simulink model "model1"  (R2021b)
settings: Solver=VariableStepAuto  StartTime=0.0  StopTime=T_end  RelTol=1e-3
values from neighbouring files (symbols this model uses):
  Te = 0.1    [ex1.m]    (also in ex3.m; ex4.m; ex5.m; ex6.m)
  u_sat = 0.5    [ex1.m]    (also in ex3.m; ex4.m; ex5.m; ex6.m)
settings Model: Creator=Michael Biselx  LastModifiedBy=Michael Biselx

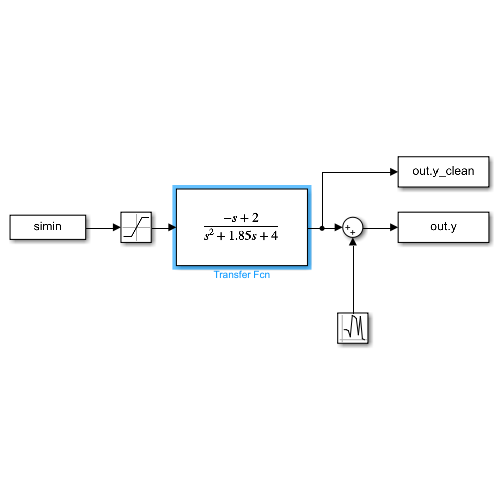
[thumbnail: Simulink's stored preview of the top-level diagram]
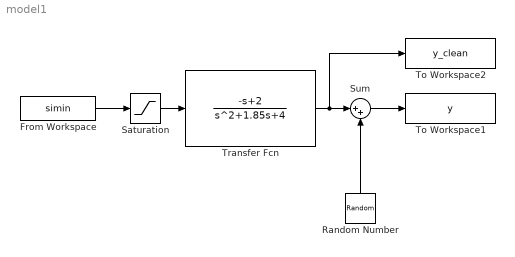
== system model1 ==
  From Workspace : FromWorkspace  VariableName=simin  SampleTime=Te
  Random Number : RandomNumber  Variance=0.01  SampleTime=Te
  Saturation : Saturate  UpperLimit=u_sat  LowerLimit=-u_sat
  Sum : Sum  Inputs=|++
  To Workspace1 : ToWorkspace  VariableName=y  SaveFormat=Timeseries  SampleTime=Te
  To Workspace2 : ToWorkspace  VariableName=y_clean  SaveFormat=Timeseries  SampleTime=Te
  Transfer Fcn : TransferFcn  Numerator=[-1 2]  Denominator=[1 1.85 4]
  wires:
  Random Number/1 -> Sum/2
  Transfer Fcn/1 -> To Workspace2/1, Sum/1
  From Workspace/1 -> Saturation/1
  Saturation/1 -> Transfer Fcn/1
  Sum/1 -> To Workspace1/1
